simulink model "cosmic_ray_system"  (R2019a)
settings: Solver=VariableStepAuto  StartTime=0.0  StopTime=1000  RelTol=1e-3
libraries: xbsIndex_r4 x6191, casper_library_misc x163, xps_library x4, casper_library_delays x4
(part 14 of 40)

== system cosmic_ray_system/cosmic_ray/coincidence_trigger/FIR1 ==
  note: reduce the number of bits arbitrarily to 18.
  note: I took a guess that the delay should be 29 because there are 25 filter coefficients plus probably 3 delays for multiplaction and 1 for addition, but this may not be exactly how it's implemented. It's not critical for it to be exact.
  bus_in : Inport
  sync_in : Inport  Port=2
  Convert{,1..63} (64 alike) : xbsIndex_r4/Convert  gui_display_data_type=Fixed-point  arith_type="Signed  (2's comp)"  n_bits=27-9  bin_pt=15-9  float_type=Single  exp_bits=8  fraction_bits=24  quantization=Truncate  overflow=Wrap  en=off  latency=0  pipeline=off  dbl_ovrd=off  block_type=convert
  Delay : xbsIndex_r4/Delay  rst=off  infoeditControl=Selection of Reset will increase slice count due to use of real FFs and instead of SRLs  en=off  latency=29  reg_retiming=off  dbl_ovrd=off  block_type=delay
  Digital FIR Filter{1..64} (64 alike) : xbsIndex_r4/Digital FIR Filter  coeff_source=off  coefficientvector=[0.000049291111379545783611425685544205066,0.012255497574972781804625299173494568095,0.085289616177628382875930412865272955969,-0.063136263203890236050952466939634177834,-0.021489412960359111082198069198057055473,-0.067555957743183181474222465112688951194,-0.017706118779731286339007567676162580028,0.080882151494431037130894424080906901509,-0.014358148251631907416081546102759602945,0.093835202832724035060252276707615237683,-0.280577771800571862392814637132687494159,-0.129748808680352711864003367736586369574,0.501393724111570460166831253445707261562,-0.129748808680352711864003367736586369574,-0.280577771800571862392814637132687494159,0.093835202832724035060252276707615237683,-0.014358148251631907416081546102759602945,0.080882151494431037130894424080906901509,-0.017706118779731286339007567676162580028,-0.067555957743183181474222465112688951194,-0.021489412960359111082198069198057055473,-0.063136263203890236050952466939634177834,0.085289616177628382875930412865272955969,0.012255497574972781804625299173494568095,0.000049291111379545783611425685544205066]  coeff_calulate=off  coefficient_width=16  coefficient_fractional_bits=15  interpolation_filter_rate=1  decimation_filter_rate=1  fda_coefficientvector=[4.92911113795458e-05 0.0122554975749728 0.0852896161776284 -0.0631362632038902 -0.0214894129603591 -0.0675559577431832 -0.0177061187797313 0.080882151494431 -0.0143581482516319 0.093835202832724 -0.280577771800572 -0.129748808680353 0.50139372411157 -0.129748808680353 -0.280577771800572 0.093835202832724 -0.0143581482516319 0.080882151494431 -0.0177061187797313 -0.0675559577431832 -0.0214894129603591 -0.0631362632038902 0.0852896161776284 0.0122554975749728 4.92911113795458e-05]  simulation_type=fast_sim  simulation_model=sysgen:fir_macro  block_type=fir_macro
  bus_create2 : Subsystem  AncestorBlock=casper_library_flow_control/bus_create  mask(bus_create){inputNum=64}
      mask prompts: inputNum "Number of inputs:"
      mask init:
      | bus_create_init(gcb,...
      |     'inputNum', inputNum);
  bus_expand : Subsystem  AncestorBlock=casper_library_flow_control/bus_expand  mask(bus_expand){mode=divisions of equal size, outputNum=64, outputWidth=10, outputBinaryPt=0, outputArithmeticType=1, show_format=off, outputToWorkspace=off, variablePrefix=out, outputToModelAsWell=on}
      mask prompts: outputNum "Number of outputs:"; outputWidth "Output width:"; outputBinaryPt "Output binary point position:"; outputArithmeticType "Output arithmetic type (ufix=0, fix=1, bool=2):"; show_format "Print format string?"; outputToWorkspace "Output to workspace?"; variablePrefix "Variable name prefix:"; outputToModelAsWell "Output to model as well?"
      mask help:
      | Expands a 'bus' made using a bus_create or Xilinx
      | concat block.
      | The input will be divided into the specified number
      | of outputs with the specified arithmetic types.
      | Divisions are made from most significant bit.
      mask init: same as cosmic_ray_system/cosmic_ray/buffer_and_packetizer/bus_expand1
      settings: AttributesFormatString=64 outputs
      mask TypeOptions mode: divisions of equal size | divisions of arbitrary size
      mask Callback mode: bus_expand_callback();
      mask Callback outputWidth: bus_expand_callback();
      mask Callback outputToWorkspace: bus_expand_callback();
  OUT : Outport
  sync_out : Outport  Port=2
  wires:
  bus_expand/63(out2) -> Digital FIR Filter60/1
  bus_expand/64(lsb_out1) -> Digital FIR Filter61/1
  Digital FIR Filter60/1 -> Convert62/1
  Digital FIR Filter61/1 -> Convert63/1
  bus_create2/1(bus_out) -> OUT/1
  sync_in/1 -> Delay/1
  bus_in/1 -> bus_expand/1(bus_in)
  Digital FIR Filter62/1 -> Convert60/1
  Digital FIR Filter29/1 -> Convert38/1
  Digital FIR Filter28/1 -> Convert23/1
  Digital FIR Filter27/1 -> Convert22/1
  bus_expand/32(out33) -> Digital FIR Filter28/1
  bus_expand/31(out34) -> Digital FIR Filter27/1
  Digital FIR Filter58/1 -> Convert61/1
  bus_expand/62(out3) -> Digital FIR Filter58/1
  bus_expand/61(out4) -> Digital FIR Filter62/1
  bus_expand/60(out5) -> Digital FIR Filter57/1
  Digital FIR Filter57/1 -> Convert51/1
  bus_expand/59(out6) -> Digital FIR Filter64/1
  Digital FIR Filter64/1 -> Convert50/1
  bus_expand/58(out7) -> Digital FIR Filter63/1
  Digital FIR Filter63/1 -> Convert49/1
  bus_expand/57(out8) -> Digital FIR Filter59/1
  Digital FIR Filter59/1 -> Convert48/1
  bus_expand/56(out9) -> Digital FIR Filter53/1
  Digital FIR Filter53/1 -> Convert47/1
  bus_expand/55(out10) -> Digital FIR Filter52/1
  Digital FIR Filter52/1 -> Convert46/1
  bus_expand/54(out11) -> Digital FIR Filter50/1
  Digital FIR Filter50/1 -> Convert45/1
  bus_expand/53(out12) -> Digital FIR Filter54/1
  Digital FIR Filter54/1 -> Convert44/1
  bus_expand/52(out13) -> Digital FIR Filter49/1
  Digital FIR Filter49/1 -> Convert43/1
  bus_expand/51(out14) -> Digital FIR Filter56/1
  Digital FIR Filter56/1 -> Convert42/1
  bus_expand/50(out15) -> Digital FIR Filter55/1
  Digital FIR Filter55/1 -> Convert59/1
  bus_expand/49(out16) -> Digital FIR Filter51/1
  Digital FIR Filter51/1 -> Convert58/1
  bus_expand/48(out17) -> Digital FIR Filter44/1
  Digital FIR Filter44/1 -> Convert57/1
  bus_expand/47(out18) -> Digital FIR Filter43/1
  Digital FIR Filter43/1 -> Convert56/1
  bus_expand/46(out19) -> Digital FIR Filter41/1
  Digital FIR Filter41/1 -> Convert55/1
  bus_expand/45(out20) -> Digital FIR Filter45/1
  Digital FIR Filter45/1 -> Convert54/1
  bus_expand/44(out21) -> Digital FIR Filter40/1
  Digital FIR Filter40/1 -> Convert53/1
  bus_expand/43(out22) -> Digital FIR Filter47/1
  Digital FIR Filter47/1 -> Convert52/1
  bus_expand/42(out23) -> Digital FIR Filter46/1
  Digital FIR Filter46/1 -> Convert41/1
  bus_expand/41(out24) -> Digital FIR Filter42/1
  Digital FIR Filter42/1 -> Convert40/1
  bus_expand/40(out25) -> Digital FIR Filter36/1
  Digital FIR Filter36/1 -> Convert31/1
  bus_expand/39(out26) -> Digital FIR Filter35/1
  Digital FIR Filter35/1 -> Convert30/1
  bus_expand/38(out27) -> Digital FIR Filter33/1
  Digital FIR Filter33/1 -> Convert29/1
  bus_expand/37(out28) -> Digital FIR Filter37/1
  Digital FIR Filter37/1 -> Convert28/1
  bus_expand/36(out29) -> Digital FIR Filter32/1
  Digital FIR Filter32/1 -> Convert27/1
  bus_expand/35(out30) -> Digital FIR Filter39/1
  Digital FIR Filter39/1 -> Convert26/1
  bus_expand/34(out31) -> Digital FIR Filter38/1
  Digital FIR Filter38/1 -> Convert25/1
  bus_expand/33(out32) -> Digital FIR Filter34/1
  Digital FIR Filter34/1 -> Convert24/1
  Digital FIR Filter25/1 -> Convert39/1
  Digital FIR Filter24/1 -> Convert37/1
  Digital FIR Filter31/1 -> Convert36/1
  Digital FIR Filter30/1 -> Convert35/1
  Digital FIR Filter26/1 -> Convert34/1
  Digital FIR Filter20/1 -> Convert33/1
  Digital FIR Filter19/1 -> Convert32/1
  Digital FIR Filter17/1 -> Convert21/1
  Digital FIR Filter21/1 -> Convert20/1
  Digital FIR Filter16/1 -> Convert19/1
  Digital FIR Filter23/1 -> Convert18/1
  Digital FIR Filter22/1 -> Convert17/1
  Digital FIR Filter18/1 -> Convert16/1
  Digital FIR Filter14/1 -> Convert15/1
  Digital FIR Filter13/1 -> Convert14/1
  Digital FIR Filter11/1 -> Convert13/1
  Digital FIR Filter15/1 -> Convert12/1
  Digital FIR Filter10/1 -> Convert11/1
  Digital FIR Filter9/1 -> Convert10/1
  Digital FIR Filter8/1 -> Convert9/1
  Digital FIR Filter12/1 -> Convert8/1
  Digital FIR Filter6/1 -> Convert7/1
  Digital FIR Filter5/1 -> Convert6/1
  Digital FIR Filter4/1 -> Convert5/1
  Digital FIR Filter7/1 -> Convert4/1
  Digital FIR Filter3/1 -> Convert3/1
  Digital FIR Filter2/1 -> Convert2/1
  Digital FIR Filter1/1 -> Convert1/1
  Digital FIR Filter48/1 -> Convert/1
  bus_expand/1(msb_out64) -> Digital FIR Filter48/1
  bus_expand/2(out63) -> Digital FIR Filter1/1
  bus_expand/3(out62) -> Digital FIR Filter2/1
  bus_expand/4(out61) -> Digital FIR Filter3/1
  bus_expand/5(out60) -> Digital FIR Filter7/1
  bus_expand/6(out59) -> Digital FIR Filter4/1
  bus_expand/7(out58) -> Digital FIR Filter5/1
  bus_expand/8(out57) -> Digital FIR Filter6/1
  bus_expand/9(out56) -> Digital FIR Filter12/1
  bus_expand/10(out55) -> Digital FIR Filter8/1
  bus_expand/11(out54) -> Digital FIR Filter9/1
  bus_expand/12(out53) -> Digital FIR Filter10/1
  bus_expand/13(out52) -> Digital FIR Filter15/1
  bus_expand/14(out51) -> Digital FIR Filter11/1
  bus_expand/15(out50) -> Digital FIR Filter13/1
  bus_expand/16(out49) -> Digital FIR Filter14/1
  bus_expand/17(out48) -> Digital FIR Filter18/1
  bus_expand/18(out47) -> Digital FIR Filter22/1
  bus_expand/19(out46) -> Digital FIR Filter23/1
  bus_expand/20(out45) -> Digital FIR Filter16/1
  bus_expand/21(out44) -> Digital FIR Filter21/1
  bus_expand/22(out43) -> Digital FIR Filter17/1
  bus_expand/23(out42) -> Digital FIR Filter19/1
  bus_expand/24(out41) -> Digital FIR Filter20/1
  bus_expand/25(out40) -> Digital FIR Filter26/1
  bus_expand/26(out39) -> Digital FIR Filter30/1
  bus_expand/27(out38) -> Digital FIR Filter31/1
  bus_expand/28(out37) -> Digital FIR Filter24/1
  bus_expand/29(out36) -> Digital FIR Filter29/1
  bus_expand/30(out35) -> Digital FIR Filter25/1
  Convert/1 -> bus_create2/1(in1)
  Convert1/1 -> bus_create2/2(in2)
  Convert2/1 -> bus_create2/3(in3)
  Convert3/1 -> bus_create2/4(in4)
  Convert4/1 -> bus_create2/5(in5)
  Convert5/1 -> bus_create2/6(in6)
  Convert6/1 -> bus_create2/7(in7)
  Convert7/1 -> bus_create2/8(in8)
  Convert8/1 -> bus_create2/9(in9)
  Convert10/1 -> bus_create2/11(in11)
  Convert11/1 -> bus_create2/12(in12)
  Convert9/1 -> bus_create2/10(in10)
  Convert17/1 -> bus_create2/18(in18)
  Convert14/1 -> bus_create2/15(in15)
  Convert16/1 -> bus_create2/17(in17)
  Convert13/1 -> bus_create2/14(in14)
  Convert12/1 -> bus_create2/13(in13)
  Convert15/1 -> bus_create2/16(in16)
  Convert21/1 -> bus_create2/22(in22)
  Convert19/1 -> bus_create2/20(in20)
  Convert22/1 -> bus_create2/31(in31)
  Convert32/1 -> bus_create2/23(in23)
  Convert39/1 -> bus_create2/30(in30)
  Convert24/1 -> bus_create2/33(in33)
  Convert36/1 -> bus_create2/27(in27)
  Convert27/1 -> bus_create2/36(in36)
  Convert35/1 -> bus_create2/26(in26)
  Convert18/1 -> bus_create2/19(in19)
  Convert33/1 -> bus_create2/24(in24)
  Convert25/1 -> bus_create2/34(in34)
  Convert34/1 -> bus_create2/25(in25)
  Convert38/1 -> bus_create2/29(in29)
  Convert20/1 -> bus_create2/21(in21)
  Convert26/1 -> bus_create2/35(in35)
  Convert37/1 -> bus_create2/28(in28)
  Convert23/1 -> bus_create2/32(in32)
  Convert57/1 -> bus_create2/48(in48)
  Convert45/1 -> bus_create2/54(in54)
  Convert54/1 -> bus_create2/45(in45)
  Convert40/1 -> bus_create2/41(in41)
  Convert28/1 -> bus_create2/37(in37)
  Convert56/1 -> bus_create2/47(in47)
  Convert31/1 -> bus_create2/40(in40)
  Convert42/1 -> bus_create2/51(in51)
  Convert41/1 -> bus_create2/42(in42)
  Convert44/1 -> bus_create2/53(in53)
  Convert59/1 -> bus_create2/50(in50)
  Convert30/1 -> bus_create2/39(in39)
  Convert29/1 -> bus_create2/38(in38)
  Convert58/1 -> bus_create2/49(in49)
  Convert52/1 -> bus_create2/43(in43)
  Convert55/1 -> bus_create2/46(in46)
  Convert43/1 -> bus_create2/52(in52)
  Convert53/1 -> bus_create2/44(in44)
  Convert50/1 -> bus_create2/59(in59)
  Convert61/1 -> bus_create2/62(in62)
  Convert46/1 -> bus_create2/55(in55)
  Convert62/1 -> bus_create2/63(in63)
  Convert49/1 -> bus_create2/58(in58)
  Delay/1 -> sync_out/1
  Convert51/1 -> bus_create2/60(in60)
  Convert47/1 -> bus_create2/56(in56)
  Convert48/1 -> bus_create2/57(in57)
  Convert63/1 -> bus_create2/64(in64)
  Convert60/1 -> bus_create2/61(in61)

== system cosmic_ray_system/cosmic_ray/coincidence_trigger/bus_threshold 1 ==
  threshold : Inport
  bus_in : Inport  Port=2
  sync_in : Inport  Port=3
  Delay7 : xbsIndex_r4/Delay  rst=off  infoeditControl=Selection of Reset will increase slice count due to use of real FFs and instead of SRLs  en=off  latency=1  reg_retiming=off  dbl_ovrd=off  block_type=delay
  Gateway Out1 : xbsIndex_r4/Gateway Out  inherit_from_input=off  hdl_port=on  rows=1  columns=1  UseAsDAC=off  DACChannel='1'  interface=None  automatic_assignment=on  address_offset=hex2dec('00')  intf_name=''  intf_description=''  timing_constraint=None  locs_specified=off  LOCs={}  io_standard={}  block_type=gatewayout
  Gateway Out2 : xbsIndex_r4/Gateway Out  inherit_from_input=off  hdl_port=on  rows=1  columns=1  UseAsDAC=off  DACChannel='1'  interface=None  automatic_assignment=on  address_offset=hex2dec('00')  intf_name=''  intf_description=''  timing_constraint=None  locs_specified=off  LOCs={}  io_standard={}  block_type=gatewayout
  Gateway Out3 : xbsIndex_r4/Gateway Out  inherit_from_input=off  hdl_port=on  rows=1  columns=1  UseAsDAC=off  DACChannel='1'  interface=None  automatic_assignment=on  address_offset=hex2dec('00')  intf_name=''  intf_description=''  timing_constraint=None  locs_specified=off  LOCs={}  io_standard={}  block_type=gatewayout
  Relational{2..65} (64 alike) : xbsIndex_r4/Relational  mode=a>b  op_type=Bool  en=off  latency=1  dbl_ovrd=off  block_type=relational
  Scope1 : Scope
  Scope2 : Scope
  Scope3 : Scope
  bus_create2 : Subsystem  AncestorBlock=casper_library_flow_control/bus_create  mask(bus_create){inputNum=64}
      mask prompts: inputNum "Number of inputs:"
      mask init:
      | bus_create_init(gcb,...
      |     'inputNum', inputNum);
  bus_expand : Subsystem  AncestorBlock=casper_library_flow_control/bus_expand  mask(bus_expand){mode=divisions of equal size, outputNum=64, outputWidth=26, outputBinaryPt=0, outputArithmeticType=1, show_format=off, outputToWorkspace=off, variablePrefix=out, outputToModelAsWell=on}
      mask prompts: outputNum "Number of outputs:"; outputWidth "Output width:"; outputBinaryPt "Output binary point position:"; outputArithmeticType "Output arithmetic type (ufix=0, fix=1, bool=2):"; show_format "Print format string?"; outputToWorkspace "Output to workspace?"; variablePrefix "Variable name prefix:"; outputToModelAsWell "Output to model as well?"
      mask help:
      | Expands a 'bus' made using a bus_create or Xilinx
      | concat block.
      | The input will be divided into the specified number
      | of outputs with the specified arithmetic types.
      | Divisions are made from most significant bit.
      mask init: same as cosmic_ray_system/cosmic_ray/buffer_and_packetizer/bus_expand1
      settings: AttributesFormatString=64 outputs
      mask TypeOptions mode: divisions of equal size | divisions of arbitrary size
      mask Callback mode: bus_expand_callback();
      mask Callback outputWidth: bus_expand_callback();
      mask Callback outputToWorkspace: bus_expand_callback();
  OUT : Outport
  sync_out : Outport  Port=2
  wires:
  Relational46/1 -> bus_create2/60(in60)
  [thresh] -> Relational61/2
  bus_expand/61(out4) -> Relational47/1
  bus_expand/45(out20) -> Relational38/1
  [thresh] -> Relational5/2
  Relational15/1 -> bus_create2/14(in14)
  bus_expand/40(out25) -> Relational65/1
  Relational36/1 -> bus_create2/43(in43)
  Relational63/1 -> bus_create2/38(in38)
  [thresh] -> Relational44/2
  Relational45/1 -> bus_create2/59(in59)
  [thresh] -> Relational23/2
  threshold/1 -> [thresh]
  Relational37/1 -> bus_create2/44(in44)
  [thresh] -> Relational7/2
  Relational53/1 -> bus_create2/51(in51)
  bus_expand/30(out35) -> Relational23/1
  bus_expand/49(out16) -> Relational51/1
  bus_expand/51(out14) -> Relational53/1
  Relational16/1 -> bus_create2/15(in15)
  bus_expand/58(out7) -> Relational43/1
  sync_in/1 -> Delay7/1
  bus_expand/53(out12) -> Relational56/1
  Relational51/1 -> bus_create2/49(in49)
  bus_expand/5(out60) -> Relational6/1
  [thresh] -> Relational33/2
  bus_expand/19(out46) -> Relational28/1
  Relational14/1 -> bus_create2/13(in13)
  Relational61/1 -> bus_create2/36(in36)
  bus_expand/44(out21) -> Relational37/1
  [thresh] -> Relational43/2
  bus_expand/37(out28) -> Relational62/1
  bus_expand/56(out9) -> Relational59/1
  Relational64/1 -> bus_create2/39(in39)
  [thresh] -> Relational56/2
  [thresh] -> Relational58/2
  [thresh] -> Relational63/2
  [thresh] -> Relational34/2
  bus_expand/29(out36) -> Relational22/1
  [thresh] -> Relational53/2
  Relational4/1 -> bus_create2/3(in3)
  [thresh] -> Relational6/2
  Relational58/1 -> bus_create2/55(in55)
  bus_expand/1(msb_out64) -> Relational2/1
  [thresh] -> Relational35/2
  bus_expand/38(out27) -> Relational63/1
  Relational35/1 -> bus_create2/42(in42)
  bus_expand/57(out8) -> Relational42/1
  Relational56/1 -> bus_create2/53(in53)
  [thresh] -> Relational28/2
  bus_expand/63(out2) -> Relational49/1
  [thresh] -> Relational10/2
  bus_expand/9(out56) -> Relational10/1
  Relational39/1 -> bus_create2/46(in46)
  bus_expand/10(out55) -> Relational11/1
  [thresh] -> Relational52/2
  [thresh] -> Relational21/2
  [thresh] -> Relational48/2
  [thresh] -> Relational32/2
  Relational59/1 -> bus_create2/56(in56)
  [thresh] -> Relational19/2
  bus_expand/21(out44) -> Relational30/1
  Relational7/1 -> bus_create2/6(in6)
  [thresh] -> Relational40/2
  bus_expand/32(out33) -> Relational25/1
  bus_expand/60(out5) -> Relational46/1
  [thresh] -> Relational24/2
  Relational3/1 -> bus_create2/2(in2)
  [thresh] -> Relational4/2
  Relational26/1 -> bus_create2/17(in17)
  [thresh] -> Relational9/2
  bus_expand/2(out63) -> Relational3/1
  [thresh] -> Relational31/2
  bus_expand/34(out31) -> Relational55/1
  [thresh] -> Relational39/2
  bus_expand/11(out54) -> Relational12/1
  bus_expand/18(out47) -> Relational27/1
  Relational22/1 -> bus_create2/29(in29)
  Relational21/1 -> bus_create2/28(in28)
  bus_expand/35(out30) -> Relational60/1
  [thresh] -> Relational22/2
  [thresh] -> Relational20/2
  [thresh] -> Relational55/2
  bus_expand/26(out39) -> Relational19/1
  [thresh] -> Relational54/2
  [thresh] -> Relational18/2
  Relational65/1 -> bus_create2/40(in40)
  Relational31/1 -> bus_create2/22(in22)
  Relational28/1 -> bus_create2/19(in19)
  bus_create2/1(bus_out) -> OUT/1
  bus_expand/33(out32) -> Relational44/1
  bus_expand/62(out3) -> Relational48/1
  [thresh] -> Relational36/2
  Delay7/1 -> sync_out/1
  [thresh] -> Relational13/2
  Relational60/1 -> bus_create2/35(in35)
  Relational49/1 -> bus_create2/63(in63)
  [thresh] -> Relational42/2
  Relational27/1 -> bus_create2/18(in18)
  [thresh] -> Relational57/2
  Relational40/1 -> bus_create2/47(in47)
  Relational19/1 -> bus_create2/26(in26)
  Relational12/1 -> bus_create2/11(in11)
  bus_expand/28(out37) -> Relational21/1
  bus_expand/41(out24) -> Relational34/1
  [thresh] -> Relational12/2
  bus_expand/16(out49) -> Relational17/1
  Relational32/1 -> bus_create2/23(in23)
  [thresh] -> Relational38/2
  Relational52/1 -> bus_create2/50(in50)
  [thresh] -> Relational3/2
  [thresh] -> Relational15/2
  bus_expand/50(out15) -> Relational52/1
  [thresh] -> Relational64/2
  bus_expand/22(out43) -> Relational31/1
  bus_expand/36(out29) -> Relational61/1
  bus_expand/46(out19) -> Relational39/1
  bus_expand/52(out13) -> Relational54/1
  Relational5/1 -> bus_create2/4(in4)
  [thresh] -> Relational45/2
  [thresh] -> Relational62/2
  bus_expand/12(out53) -> Relational13/1
  [thresh] -> Relational16/2
  bus_expand/8(out57) -> Relational9/1
  [thresh] -> Relational59/2
  bus_expand/7(out58) -> Relational8/1
  bus_expand/3(out62) -> Relational4/1
  [thresh] -> Relational25/2
  bus_expand/20(out45) -> Relational29/1
  Relational9/1 -> bus_create2/8(in8)
  bus_expand/15(out50) -> Relational16/1
  bus_expand/48(out17) -> Relational41/1
  Relational54/1 -> bus_create2/52(in52)
  [thresh] -> Relational29/2
  Relational44/1 -> bus_create2/33(in33)
  Relational43/1 -> bus_create2/58(in58)
  bus_expand/4(out61) -> Relational5/1
  [thresh] -> Relational14/2
  bus_expand/13(out52) -> Relational14/1
  Relational50/1 -> Gateway Out1/1, bus_create2/64(in64)
  [thresh] -> Relational8/2
  bus_expand/43(out22) -> Relational36/1
  Relational25/1 -> bus_create2/32(in32)
  Relational33/1 -> bus_create2/24(in24)
  Relational29/1 -> bus_create2/20(in20)
  [thresh] -> Relational30/2
  [thresh] -> Relational17/2
  [thresh] -> Relational60/2
  bus_expand/39(out26) -> Relational64/1
  [thresh] -> Relational49/2
  Relational30/1 -> bus_create2/21(in21)
  bus_in/1 -> bus_expand/1(bus_in)
  [thresh] -> Relational46/2
  bus_expand/31(out34) -> Relational24/1
  Relational41/1 -> bus_create2/48(in48)
  [thresh] -> Relational37/2
  Relational38/1 -> bus_create2/45(in45)
  bus_expand/17(out48) -> Relational26/1
  bus_expand/27(out38) -> Relational20/1
  bus_expand/23(out42) -> Relational32/1
  bus_expand/55(out10) -> Relational58/1
  Relational8/1 -> bus_create2/7(in7)
  Relational20/1 -> bus_create2/27(in27)
  Relational17/1 -> bus_create2/16(in16)
  Relational42/1 -> bus_create2/57(in57)
  Relational55/1 -> bus_create2/34(in34)
  [thresh] -> Relational11/2
  Relational23/1 -> bus_create2/30(in30)
  Relational18/1 -> bus_create2/25(in25)
  Relational48/1 -> bus_create2/62(in62)
  Relational10/1 -> bus_create2/9(in9)
  Relational62/1 -> bus_create2/37(in37)
  Relational24/1 -> bus_create2/31(in31)
  [thresh] -> Relational47/2
  [thresh] -> Relational27/2
  bus_expand/47(out18) -> Relational40/1
  [thresh] -> Relational51/2
  bus_expand/6(out59) -> Relational7/1
  [thresh] -> Relational26/2
  Relational2/1 -> bus_create2/1(in1)
  [thresh] -> Relational65/2
  Relational11/1 -> bus_create2/10(in10)
  Relational13/1 -> bus_create2/12(in12)
  [thresh] -> Relational41/2
  Relational34/1 -> bus_create2/41(in41)
  Relational57/1 -> bus_create2/54(in54)
  bus_expand/54(out11) -> Relational57/1
  bus_expand/59(out6) -> Relational45/1
  Relational6/1 -> bus_create2/5(in5)
  bus_expand/42(out23) -> Relational35/1
  [thresh] -> Relational2/2
  bus_expand/14(out51) -> Relational15/1
  bus_expand/25(out40) -> Relational18/1
  bus_expand/24(out41) -> Relational33/1
  Relational47/1 -> bus_create2/61(in61)
  Gateway Out1/1 -> Scope1/1
  Gateway Out2/1 -> Scope2/1
  [thresh] -> Gateway Out2/1, Relational50/2
  bus_expand/64(lsb_out1) -> Gateway Out3/1, Relational50/1
  Gateway Out3/1 -> Scope3/1

== system cosmic_ray_system/cosmic_ray/coincidence_trigger/bus_threshold 2 ==
  threshold : Inport
  bus_in : Inport  Port=2
  sync_in : Inport  Port=3
  Delay7 : xbsIndex_r4/Delay  rst=off  infoeditControl=Selection of Reset will increase slice count due to use of real FFs and instead of SRLs  en=off  latency=1  reg_retiming=off  dbl_ovrd=off  block_type=delay
  Relational{2..65} (64 alike) : xbsIndex_r4/Relational  mode=a>b  op_type=Bool  en=off  latency=1  dbl_ovrd=off  block_type=relational
  bus_create2 : Subsystem  AncestorBlock=casper_library_flow_control/bus_create  mask(bus_create){inputNum=64}
      mask prompts: inputNum "Number of inputs:"
      mask init:
      | bus_create_init(gcb,...
      |     'inputNum', inputNum);
  bus_expand : Subsystem  AncestorBlock=casper_library_flow_control/bus_expand  mask(bus_expand){mode=divisions of equal size, outputNum=64, outputWidth=26, outputBinaryPt=0, outputArithmeticType=1, show_format=off, outputToWorkspace=off, variablePrefix=out, outputToModelAsWell=on}
      mask prompts: outputNum "Number of outputs:"; outputWidth "Output width:"; outputBinaryPt "Output binary point position:"; outputArithmeticType "Output arithmetic type (ufix=0, fix=1, bool=2):"; show_format "Print format string?"; outputToWorkspace "Output to workspace?"; variablePrefix "Variable name prefix:"; outputToModelAsWell "Output to model as well?"
      mask help:
      | Expands a 'bus' made using a bus_create or Xilinx
      | concat block.
      | The input will be divided into the specified number
      | of outputs with the specified arithmetic types.
      | Divisions are made from most significant bit.
      mask init: same as cosmic_ray_system/cosmic_ray/buffer_and_packetizer/bus_expand1
      settings: AttributesFormatString=64 outputs
      mask TypeOptions mode: divisions of equal size | divisions of arbitrary size
      mask Callback mode: bus_expand_callback();
      mask Callback outputWidth: bus_expand_callback();
      mask Callback outputToWorkspace: bus_expand_callback();
  OUT : Outport
  sync_out : Outport  Port=2
  wires:
  bus_expand/24(out41) -> Relational33/1
  bus_expand/25(out40) -> Relational18/1
  bus_expand/14(out51) -> Relational15/1
  [thresh] -> Relational2/2
  bus_expand/42(out23) -> Relational35/1
  Relational6/1 -> bus_create2/5(in5)
  bus_expand/59(out6) -> Relational45/1
  bus_expand/54(out11) -> Relational57/1
  Relational57/1 -> bus_create2/54(in54)
  Relational34/1 -> bus_create2/41(in41)
  [thresh] -> Relational41/2
  Relational13/1 -> bus_create2/12(in12)
  Relational11/1 -> bus_create2/10(in10)
  [thresh] -> Relational65/2
  Relational2/1 -> bus_create2/1(in1)
  [thresh] -> Relational26/2
  bus_expand/6(out59) -> Relational7/1
  [thresh] -> Relational51/2
  bus_expand/47(out18) -> Relational40/1
  [thresh] -> Relational27/2
  [thresh] -> Relational47/2
  Relational24/1 -> bus_create2/31(in31)
  Relational62/1 -> bus_create2/37(in37)
  Relational10/1 -> bus_create2/9(in9)
  Relational48/1 -> bus_create2/62(in62)
  Relational18/1 -> bus_create2/25(in25)
  Relational23/1 -> bus_create2/30(in30)
  [thresh] -> Relational11/2
  Relational55/1 -> bus_create2/34(in34)
  Relational42/1 -> bus_create2/57(in57)
  Relational17/1 -> bus_create2/16(in16)
  Relational20/1 -> bus_create2/27(in27)
  Relational8/1 -> bus_create2/7(in7)
  bus_expand/55(out10) -> Relational58/1
  bus_expand/23(out42) -> Relational32/1
  bus_expand/27(out38) -> Relational20/1
  bus_expand/17(out48) -> Relational26/1
  Relational38/1 -> bus_create2/45(in45)
  [thresh] -> Relational37/2
  Relational41/1 -> bus_create2/48(in48)
  bus_expand/31(out34) -> Relational24/1
  [thresh] -> Relational46/2
  bus_in/1 -> bus_expand/1(bus_in)
  Relational30/1 -> bus_create2/21(in21)
  [thresh] -> Relational49/2
  bus_expand/39(out26) -> Relational64/1
  [thresh] -> Relational60/2
  [thresh] -> Relational17/2
  [thresh] -> Relational30/2
  Relational29/1 -> bus_create2/20(in20)
  Relational33/1 -> bus_create2/24(in24)
  Relational25/1 -> bus_create2/32(in32)
  bus_expand/43(out22) -> Relational36/1
  [thresh] -> Relational8/2
  Relational50/1 -> bus_create2/64(in64)
  bus_expand/13(out52) -> Relational14/1
  [thresh] -> Relational14/2
  bus_expand/4(out61) -> Relational5/1
  Relational43/1 -> bus_create2/58(in58)
  Relational44/1 -> bus_create2/33(in33)
  [thresh] -> Relational29/2
  Relational54/1 -> bus_create2/52(in52)
  bus_expand/48(out17) -> Relational41/1
  bus_expand/15(out50) -> Relational16/1
  Relational9/1 -> bus_create2/8(in8)
  bus_expand/20(out45) -> Relational29/1
  [thresh] -> Relational25/2
  bus_expand/3(out62) -> Relational4/1
  bus_expand/7(out58) -> Relational8/1
  [thresh] -> Relational59/2
  bus_expand/8(out57) -> Relational9/1
  [thresh] -> Relational16/2
  bus_expand/12(out53) -> Relational13/1
  [thresh] -> Relational62/2
  [thresh] -> Relational45/2
  Relational5/1 -> bus_create2/4(in4)
  bus_expand/52(out13) -> Relational54/1
  bus_expand/46(out19) -> Relational39/1
  bus_expand/36(out29) -> Relational61/1
  bus_expand/22(out43) -> Relational31/1
  [thresh] -> Relational64/2
  bus_expand/50(out15) -> Relational52/1
  [thresh] -> Relational15/2
  [thresh] -> Relational3/2
  Relational52/1 -> bus_create2/50(in50)
  [thresh] -> Relational38/2
  Relational32/1 -> bus_create2/23(in23)
  bus_expand/16(out49) -> Relational17/1
  [thresh] -> Relational12/2
  bus_expand/41(out24) -> Relational34/1
  bus_expand/28(out37) -> Relational21/1
  Relational12/1 -> bus_create2/11(in11)
  Relational19/1 -> bus_create2/26(in26)
  Relational40/1 -> bus_create2/47(in47)
  [thresh] -> Relational57/2
  Relational27/1 -> bus_create2/18(in18)
  [thresh] -> Relational42/2
  Relational49/1 -> bus_create2/63(in63)
  Relational60/1 -> bus_create2/35(in35)
  [thresh] -> Relational13/2
  Delay7/1 -> sync_out/1
  [thresh] -> Relational36/2
  bus_expand/62(out3) -> Relational48/1
  bus_expand/33(out32) -> Relational44/1
  bus_create2/1(bus_out) -> OUT/1
  Relational28/1 -> bus_create2/19(in19)
  Relational31/1 -> bus_create2/22(in22)
  Relational65/1 -> bus_create2/40(in40)
  [thresh] -> Relational18/2
  [thresh] -> Relational54/2
  bus_expand/26(out39) -> Relational19/1
  [thresh] -> Relational55/2
  [thresh] -> Relational20/2
  [thresh] -> Relational22/2
  bus_expand/35(out30) -> Relational60/1
  Relational21/1 -> bus_create2/28(in28)
  Relational22/1 -> bus_create2/29(in29)
  bus_expand/18(out47) -> Relational27/1
  bus_expand/11(out54) -> Relational12/1
  [thresh] -> Relational39/2
  bus_expand/34(out31) -> Relational55/1
  [thresh] -> Relational31/2
  bus_expand/2(out63) -> Relational3/1
  [thresh] -> Relational9/2
  Relational26/1 -> bus_create2/17(in17)
  [thresh] -> Relational4/2
  Relational3/1 -> bus_create2/2(in2)
  [thresh] -> Relational24/2
  bus_expand/60(out5) -> Relational46/1
  bus_expand/32(out33) -> Relational25/1
  [thresh] -> Relational40/2
  Relational7/1 -> bus_create2/6(in6)
  bus_expand/21(out44) -> Relational30/1
  [thresh] -> Relational19/2
  Relational59/1 -> bus_create2/56(in56)
  [thresh] -> Relational32/2
  [thresh] -> Relational48/2
  [thresh] -> Relational21/2
  [thresh] -> Relational52/2
  bus_expand/10(out55) -> Relational11/1
  Relational39/1 -> bus_create2/46(in46)
  bus_expand/9(out56) -> Relational10/1
  [thresh] -> Relational10/2
  bus_expand/63(out2) -> Relational49/1
  [thresh] -> Relational28/2
  Relational56/1 -> bus_create2/53(in53)
  bus_expand/57(out8) -> Relational42/1
  [thresh] -> Relational50/2
  Relational35/1 -> bus_create2/42(in42)
  bus_expand/38(out27) -> Relational63/1
  [thresh] -> Relational35/2
  bus_expand/1(msb_out64) -> Relational2/1
  Relational58/1 -> bus_create2/55(in55)
  [thresh] -> Relational6/2
  bus_expand/64(lsb_out1) -> Relational50/1
  Relational4/1 -> bus_create2/3(in3)
  [thresh] -> Relational53/2
  bus_expand/29(out36) -> Relational22/1
  [thresh] -> Relational34/2
  [thresh] -> Relational63/2
  [thresh] -> Relational58/2
  [thresh] -> Relational56/2
  Relational64/1 -> bus_create2/39(in39)
  bus_expand/56(out9) -> Relational59/1
  bus_expand/37(out28) -> Relational62/1
  [thresh] -> Relational43/2
  bus_expand/44(out21) -> Relational37/1
  Relational61/1 -> bus_create2/36(in36)
  Relational47/1 -> bus_create2/61(in61)
  Relational14/1 -> bus_create2/13(in13)
  bus_expand/19(out46) -> Relational28/1
  [thresh] -> Relational33/2
  bus_expand/5(out60) -> Relational6/1
  Relational51/1 -> bus_create2/49(in49)
  bus_expand/53(out12) -> Relational56/1
  sync_in/1 -> Delay7/1
  bus_expand/58(out7) -> Relational43/1
  Relational16/1 -> bus_create2/15(in15)
  bus_expand/51(out14) -> Relational53/1
  bus_expand/49(out16) -> Relational51/1
  bus_expand/30(out35) -> Relational23/1
  Relational53/1 -> bus_create2/51(in51)
  [thresh] -> Relational7/2
  Relational37/1 -> bus_create2/44(in44)
  threshold/1 -> [thresh]
  [thresh] -> Relational23/2
  Relational45/1 -> bus_create2/59(in59)
  [thresh] -> Relational44/2
  Relational63/1 -> bus_create2/38(in38)
  Relational36/1 -> bus_create2/43(in43)
  bus_expand/40(out25) -> Relational65/1
  Relational15/1 -> bus_create2/14(in14)
  [thresh] -> Relational5/2
  bus_expand/45(out20) -> Relational38/1
  bus_expand/61(out4) -> Relational47/1
  [thresh] -> Relational61/2
  Relational46/1 -> bus_create2/60(in60)

== system cosmic_ray_system/cosmic_ray/coincidence_trigger/custom_pulse_extend_with_sync_no_edgedetect  ==
  note: Add one so that the actual length of the extended pulse is the input number of clock cycles. Note that for the version with the edge detect I had to subtract one here.
  "in " : Inport
  "pulse_length " : Inport  Port=2
  sync_in : Inport  Port=3
  AddSub1 : xbsIndex_r4/AddSub  mode=Addition  use_carryin=off  use_carryout=off  en=off  latency=1  precision=Full  arith_type=Unsigned  n_bits=16  bin_pt=14  quantization=Truncate  overflow=Wrap  use_behavioral_HDL=on  hw_selection=Fabric  pipelined=off  dbl_ovrd=off  block_type=addsub
  Constant1 : xbsIndex_r4/Constant  const=1  gui_display_data_type=Fixed-point  arith_type=Unsigned  n_bits=1  bin_pt=0  preci_type=Single  exp_width=8  frac_width=24  explicit_period=on  period=1  equ=P=C  opselect=C  inp2=PCIN>>17  opr=+  inp1=P  carry=CIN  dbl_ovrd=off  block_type=constant
  Counter : xbsIndex_r4/Counter  cnt_type=Free Running  cnt_to=Inf  operation=Up  start_count=0  cnt_by_val=1  arith_type=Unsigned  n_bits=12  bin_pt=0  load_pin=off  rst=on  en=on  explicit_period=on  period=1  use_behavioral_HDL=off  implementation=Fabric  dbl_ovrd=off  block_type=counter
  Delay1 : xbsIndex_r4/Delay  rst=off  infoeditControl=Selection of Reset will increase slice count due to use of real FFs and instead of SRLs  en=off  latency=2  reg_retiming=off  dbl_ovrd=off  block_type=delay
  Relational : xbsIndex_r4/Relational  mode=a<b  op_type=Bool  en=off  latency=1  dbl_ovrd=off  block_type=relational
  "out " : Outport
  sync_out : Outport  Port=2
  wires:
  Counter/1 -> Relational/1
  Delay1/1 -> sync_out/1
  "in "/1 -> Counter/1
  sync_in/1 -> Delay1/1
  Relational/1 -> "out "/1, Counter/2
  Constant1/1 -> AddSub1/2
  AddSub1/1 -> Relational/2
  "pulse_length "/1 -> AddSub1/1

== system cosmic_ray_system/cosmic_ray/coincidence_trigger/square_bus_components ==
  IN : Inport
  sync_in : Inport  Port=2
  Delay7 : xbsIndex_r4/Delay  rst=off  infoeditControl=Selection of Reset will increase slice count due to use of real FFs and instead of SRLs  en=off  latency=3  reg_retiming=off  dbl_ovrd=off  block_type=delay
  Gateway Out : xbsIndex_r4/Gateway Out  inherit_from_input=off  hdl_port=off  rows=1  columns=1  UseAsDAC=off  DACChannel='1'  interface=None  automatic_assignment=on  address_offset=hex2dec('00')  intf_name=''  intf_description=''  timing_constraint=None  locs_specified=off  LOCs={}  io_standard={}  block_type=gatewayout
  Gateway Out1 : xbsIndex_r4/Gateway Out  inherit_from_input=off  hdl_port=off  rows=1  columns=1  UseAsDAC=off  DACChannel='1'  interface=None  automatic_assignment=on  address_offset=hex2dec('00')  intf_name=''  intf_description=''  timing_constraint=None  locs_specified=off  LOCs={}  io_standard={}  block_type=gatewayout
  Scope : Scope
  Scope1 : Scope
  Scope{2..5} (4 alike) : Scope  Commented=on
  Subsystem : Subsystem
  Subsystem1 : Subsystem
  Subsystem10 : Subsystem
  Subsystem11 : Subsystem
  Subsystem12 : Subsystem
  Subsystem13 : Subsystem
  Subsystem14 : Subsystem
  Subsystem15 : Subsystem
  Subsystem16 : Subsystem
  Subsystem17 : Subsystem
  Subsystem18 : Subsystem
  Subsystem19 : Subsystem
  Subsystem2 : Subsystem
  Subsystem20 : Subsystem
  Subsystem21 : Subsystem
  Subsystem22 : Subsystem
  Subsystem23 : Subsystem
  Subsystem24 : Subsystem
  Subsystem25 : Subsystem
  Subsystem26 : Subsystem
  Subsystem27 : Subsystem
  Subsystem28 : Subsystem
  Subsystem29 : Subsystem
  Subsystem3 : Subsystem
  Subsystem30 : Subsystem
  Subsystem31 : Subsystem
  Subsystem32 : Subsystem
  Subsystem33 : Subsystem
  Subsystem34 : Subsystem
  Subsystem35 : Subsystem
  Subsystem36 : Subsystem
  Subsystem37 : Subsystem
  Subsystem38 : Subsystem
  Subsystem39 : Subsystem
  Subsystem4 : Subsystem
  Subsystem40 : Subsystem
  Subsystem41 : Subsystem
  Subsystem42 : Subsystem
  Subsystem43 : Subsystem
  Subsystem44 : Subsystem
  Subsystem45 : Subsystem
  Subsystem46 : Subsystem
  Subsystem47 : Subsystem
  Subsystem48 : Subsystem
  Subsystem49 : Subsystem
  Subsystem5 : Subsystem
  Subsystem50 : Subsystem
  Subsystem51 : Subsystem
  Subsystem52 : Subsystem
  Subsystem53 : Subsystem
  Subsystem54 : Subsystem
  Subsystem55 : Subsystem
  Subsystem56 : Subsystem
  Subsystem57 : Subsystem
  Subsystem58 : Subsystem
  Subsystem59 : Subsystem
  Subsystem6 : Subsystem
  Subsystem60 : Subsystem
  Subsystem61 : Subsystem
  Subsystem62 : Subsystem
  Subsystem63 : Subsystem
  Subsystem7 : Subsystem
  Subsystem8 : Subsystem
  Subsystem9 : Subsystem
  bus_create2 : Subsystem  AncestorBlock=casper_library_flow_control/bus_create  mask(bus_create){inputNum=64}
      mask prompts: inputNum "Number of inputs:"
      mask init:
      | bus_create_init(gcb,...
      |     'inputNum', inputNum);
  bus_expand : Subsystem  AncestorBlock=casper_library_flow_control/bus_expand  mask(bus_expand){mode=divisions of equal size, outputNum=64, outputWidth=18, outputBinaryPt=6, outputArithmeticType=1, show_format=off, outputToWorkspace=off, variablePrefix=out, outputToModelAsWell=on}
      mask prompts: outputNum "Number of outputs:"; outputWidth "Output width:"; outputBinaryPt "Output binary point position:"; outputArithmeticType "Output arithmetic type (ufix=0, fix=1, bool=2):"; show_format "Print format string?"; outputToWorkspace "Output to workspace?"; variablePrefix "Variable name prefix:"; outputToModelAsWell "Output to model as well?"
      mask help:
      | Expands a 'bus' made using a bus_create or Xilinx
      | concat block.
      | The input will be divided into the specified number
      | of outputs with the specified arithmetic types.
      | Divisions are made from most significant bit.
      mask init: same as cosmic_ray_system/cosmic_ray/buffer_and_packetizer/bus_expand1
      settings: AttributesFormatString=64 outputs
      mask TypeOptions mode: divisions of equal size | divisions of arbitrary size
      mask Callback mode: bus_expand_callback();
      mask Callback outputWidth: bus_expand_callback();
      mask Callback outputToWorkspace: bus_expand_callback();
  OUT : Outport
  sync_out : Outport  Port=2
  wires:
  Delay7/1 -> sync_out/1
  sync_in/1 -> Delay7/1
  IN/1 -> bus_expand/1(bus_in)
  bus_create2/1(bus_out) -> OUT/1
  Gateway Out/1 -> Scope/1
  Gateway Out1/1 -> Scope1/1
  Subsystem/1(out) -> Gateway Out/1, bus_create2/1(in1)
  bus_expand/1(msb_out64) -> Subsystem/1(in)
  Subsystem1/1(out) -> Gateway Out1/1, bus_create2/2(in2)
  Subsystem2/1(out) -> bus_create2/3(in3)
  Subsystem3/1(out) -> bus_create2/4(in4)
  Subsystem4/1(out) -> bus_create2/5(in5)
  Subsystem5/1(out) -> bus_create2/6(in6)
  Subsystem6/1(out) -> bus_create2/7(in7)
  Subsystem7/1(out) -> bus_create2/8(in8)
  Subsystem8/1(out) -> bus_create2/9(in9)
  Subsystem9/1(out) -> bus_create2/10(in10)
  Subsystem10/1(out) -> bus_create2/11(in11)
  Subsystem11/1(out) -> bus_create2/12(in12)
  Subsystem12/1(out) -> bus_create2/13(in13)
  Subsystem13/1(out) -> bus_create2/14(in14)
  Subsystem14/1(out) -> bus_create2/15(in15)
  Subsystem15/1(out) -> bus_create2/16(in16)
  Subsystem16/1(out) -> bus_create2/17(in17)
  Subsystem17/1(out) -> bus_create2/18(in18)
  Subsystem24/1(out) -> bus_create2/19(in19)
  Subsystem25/1(out) -> bus_create2/20(in20)
  Subsystem26/1(out) -> bus_create2/21(in21)
  Subsystem27/1(out) -> bus_create2/22(in22)
  Subsystem28/1(out) -> bus_create2/23(in23)
  Subsystem29/1(out) -> bus_create2/24(in24)
  Subsystem30/1(out) -> bus_create2/25(in25)
  Subsystem31/1(out) -> bus_create2/26(in26)
  Subsystem18/1(out) -> bus_create2/27(in27)
  Subsystem19/1(out) -> bus_create2/28(in28)
  Subsystem20/1(out) -> bus_create2/29(in29)
  Subsystem21/1(out) -> bus_create2/30(in30)
  Subsystem22/1(out) -> bus_create2/31(in31)
  Subsystem23/1(out) -> bus_create2/32(in32)
  Subsystem32/1(out) -> bus_create2/33(in33)
  Subsystem33/1(out) -> bus_create2/34(in34)
  Subsystem40/1(out) -> bus_create2/35(in35)
  Subsystem41/1(out) -> bus_create2/36(in36)
  Subsystem42/1(out) -> bus_create2/37(in37)
  Subsystem43/1(out) -> bus_create2/38(in38)
  Subsystem44/1(out) -> bus_create2/39(in39)
  Subsystem45/1(out) -> bus_create2/40(in40)
  Subsystem46/1(out) -> bus_create2/41(in41)
  Subsystem47/1(out) -> bus_create2/42(in42)
  Subsystem34/1(out) -> bus_create2/43(in43)
  Subsystem35/1(out) -> bus_create2/44(in44)
  Subsystem36/1(out) -> bus_create2/45(in45)
  Subsystem37/1(out) -> bus_create2/46(in46)
  Subsystem38/1(out) -> bus_create2/47(in47)
  Subsystem39/1(out) -> bus_create2/48(in48)
  Subsystem48/1(out) -> bus_create2/49(in49)
  Subsystem49/1(out) -> bus_create2/50(in50)
  Subsystem56/1(out) -> bus_create2/51(in51)
  Subsystem57/1(out) -> bus_create2/52(in52)
  Subsystem58/1(out) -> bus_create2/53(in53)
  Subsystem59/1(out) -> bus_create2/54(in54)
  Subsystem60/1(out) -> bus_create2/55(in55)
  Subsystem61/1(out) -> bus_create2/56(in56)
  Subsystem62/1(out) -> bus_create2/57(in57)
  Subsystem63/1(out) -> bus_create2/58(in58)
  Subsystem50/1(out) -> bus_create2/59(in59)
  Subsystem51/1(out) -> bus_create2/60(in60)
  Subsystem52/1(out) -> bus_create2/61(in61)
  Subsystem53/1(out) -> bus_create2/62(in62)
  Subsystem54/1(out) -> bus_create2/63(in63)
  Subsystem55/1(out) -> bus_create2/64(in64)
  bus_expand/2(out63) -> Subsystem1/1(in)
  bus_expand/3(out62) -> Subsystem2/1(in)
  bus_expand/4(out61) -> Subsystem3/1(in)
  bus_expand/5(out60) -> Subsystem4/1(in)
  bus_expand/6(out59) -> Subsystem5/1(in)
  bus_expand/7(out58) -> Subsystem6/1(in)
  bus_expand/8(out57) -> Subsystem7/1(in)
  bus_expand/9(out56) -> Subsystem8/1(in)
  bus_expand/10(out55) -> Subsystem9/1(in)
  bus_expand/11(out54) -> Subsystem10/1(in)
  bus_expand/12(out53) -> Subsystem11/1(in)
  bus_expand/13(out52) -> Subsystem12/1(in)
  bus_expand/14(out51) -> Subsystem13/1(in)
  bus_expand/15(out50) -> Subsystem14/1(in)
  bus_expand/16(out49) -> Subsystem15/1(in)
  bus_expand/17(out48) -> Subsystem16/1(in)
  bus_expand/18(out47) -> Subsystem17/1(in)
  bus_expand/19(out46) -> Subsystem24/1(in)
  bus_expand/20(out45) -> Subsystem25/1(in)
  bus_expand/21(out44) -> Subsystem26/1(in)
  bus_expand/22(out43) -> Subsystem27/1(in)
  bus_expand/23(out42) -> Subsystem28/1(in)
  bus_expand/24(out41) -> Subsystem29/1(in)
  bus_expand/25(out40) -> Subsystem30/1(in)
  bus_expand/26(out39) -> Subsystem31/1(in)
  bus_expand/27(out38) -> Subsystem18/1(in)
  bus_expand/28(out37) -> Subsystem19/1(in)
  bus_expand/29(out36) -> Subsystem20/1(in)
  bus_expand/30(out35) -> Subsystem21/1(in)
  bus_expand/31(out34) -> Subsystem22/1(in)
  bus_expand/32(out33) -> Subsystem23/1(in)
  bus_expand/33(out32) -> Subsystem32/1(in)
  bus_expand/34(out31) -> Subsystem33/1(in)
  bus_expand/35(out30) -> Subsystem40/1(in)
  bus_expand/36(out29) -> Subsystem41/1(in)
  bus_expand/37(out28) -> Subsystem42/1(in)
  bus_expand/38(out27) -> Subsystem43/1(in)
  bus_expand/39(out26) -> Subsystem44/1(in)
  bus_expand/40(out25) -> Subsystem45/1(in)
  bus_expand/41(out24) -> Subsystem46/1(in)
  bus_expand/42(out23) -> Subsystem47/1(in)
  bus_expand/43(out22) -> Subsystem34/1(in)
  bus_expand/44(out21) -> Subsystem35/1(in)
  bus_expand/45(out20) -> Subsystem36/1(in)
  bus_expand/46(out19) -> Subsystem37/1(in)
  bus_expand/47(out18) -> Subsystem38/1(in)
  bus_expand/48(out17) -> Subsystem39/1(in)
  bus_expand/49(out16) -> Subsystem48/1(in)
  bus_expand/50(out15) -> Subsystem49/1(in)
  bus_expand/51(out14) -> Subsystem56/1(in)
  bus_expand/52(out13) -> Subsystem57/1(in)
  bus_expand/53(out12) -> Subsystem58/1(in)
  bus_expand/54(out11) -> Subsystem59/1(in)
  bus_expand/55(out10) -> Subsystem60/1(in)
  bus_expand/56(out9) -> Subsystem61/1(in)
  bus_expand/57(out8) -> Subsystem62/1(in)
  bus_expand/58(out7) -> Subsystem63/1(in)
  bus_expand/59(out6) -> Subsystem50/1(in)
  bus_expand/60(out5) -> Subsystem51/1(in)
  bus_expand/61(out4) -> Subsystem52/1(in)
  bus_expand/62(out3) -> Subsystem53/1(in)
  bus_expand/63(out2) -> Subsystem54/1(in)
  bus_expand/64(lsb_out1) -> Subsystem55/1(in)
